simulink model "roll_control"  (R2020b)
settings: Solver=VariableStepAuto  StartTime=0.0  StopTime=3.45  FixedStep=0.001  RelTol=1e-5  AbsTol=1e-6
PostLoadFcn:
  | path = fileparts(which(bdroot))
  | cd(path)
  | masscgI = xlsread('mass,cg,I','mass,cg,I');
  | ThrustTable = xlsread('F15_Thrust','Sheet1');
  | u = xlsread('../../scp_new_problem/src/u.csv','u');
InitFcn:
  | HeightAboveSeaLevel = 5.4419142084;
  | 
  | GustStart = 1;
  | GustLength = [120, 130, 80];
  | GuestAmplitude = [ 2.5, -2.5,  1];
  | 
  | ShearSpeed = 4;
  | ShearDirection = 75;
  | 
  | Croll = 0.001 * (rand - 0.5);
  | Cyaw = 0.05 * (rand - 0.5);
  | Cside = 0.001 * (rand - 0.5);
  | 
  | GustStart = 2 * rand;
  | GustLength = [100 + 50 * (rand - 0.5), 100 + 50 * (rand - 0.5), 100 + 50 * (rand - 0.5)];
  | GuestAmplitude = [ 5 * (rand - 0.5), 5 * (rand - 0.5),  5 * (rand - 0.5)];
  | 
  | ShearSpeed = 5 * rand;
  | ShearDirection = 360 * rand;
  | 
  | HeightAboveSeaLevel = rand * 1000;
values from neighbouring files (symbols this model uses):
  cg = temp(4)    [NonlinearStateEstimationForActuatorDelay.m]
  D = zeros(size(B))    [RocketOutputFunction.m]    (also in StateSpaceController.m; TimeDelayCompensationElevator.m = [0; 0])
  F = eye(6)    [MEKFAttitudeOnly.m]
  I = reshape(x(1:9), [3 3])    [AdaptiveLQR.m]    (also in MEKF.m = diag([0.08 0.08 0.002]); MEKFAttitudeOnly.m = diag([0.08 0.08 0.002]); MEKF_old.m = diag([0.08 0.08 0.002]); NonlinearStateEstimationForActuatorDelay.m = diag([Ixx, Ixx, Izz]))
  K = 1.1    [DATCOMvsOR.m]    (also in Forces_and_Moments_Calculator.m; MEKF.m = (P * H.') / (H * P * H.' + V); MEKFAttitudeOnly.m = P2 * H' * inv(S); MEKF_old.m = (P * H.') / (H * P * H.' + V))
  mass = 1.0565    [ImpactVelocityNotParallelMatlab.m]    (also in NonlinearStateEstimationForActuatorDelay.m = temp(1); OneDLanding.m; RunImpactVelocityParforCompiled.m; StateSpaceController.m = 1.0616753546)
  q = x(13:16)    [AdaptiveLQR.m]    (also in MEKF.m = nominal_state(4:7); MEKFAttitudeOnly.m = [1 0 0 0]; MEKF_old.m = nominal_state(4:7); NonlinearStateEstimationForActuatorDelay.m = x(4:7))
  r = [0; 0; -(rocket_length - Average_cg)]    [StateSpaceController.m]    (also in TimeDelayCompensationElevator.m = [0;0]; Tracker.m)
  s = linspace(0, 100, nums)    [ImpactVelocityFunction.m]    (also in ImpactVelocityNotParallelMatlab.m = 1:5:500; ParallelImpactVelocity.m = .1:.01:500; ParralelRun.m = linspace(5,7, nums); RunImpactVelocityParforCompiled.m = 1:0.1:500)
  whentoignite = [s(row); v(col)]    [SecondPartLandingAlgorithm.m]
undefined symbols (not defined in the file or in its folder): Angle, Axis, deg, e0_0, e1_0, e2_0, e3_0, Earth, Kri, Light, magnitude, MIL, rad, WGS84
libraries: aerolibutil x7, vrlib x6, shared6dof x6, aerolibconvert2 x5, simulink x4, sharedtransform x4, aerolibwind2 x3, pid_lib x3, robotcorelib x2, sharedutil x2, aerolibasang x2, aerolibatmos2 x1
(part 2 of 3)

== system roll_control/Subsystem/Acceleration Calculator/Aero Forces and Moments ==
  Mach : Inport
  Local Airspeed (m/s) : Inport  Port=2
  AoA (rad) : Inport  Port=3
  Density : Inport  Port=4
  Temperature : Inport  Port=5
  Dynamic Pressure : Inport  Port=6
  Center of Mass X : Inport  Port=7
  Angular velocity (rad/s) : Inport  Port=8
  Axial Drag Calculator : Subsystem
  CN and Cm calculator : Subsystem
  Coefficients to Force : Subsystem
  Coefficients to Moment : Subsystem
  Constants : Subsystem
  Croll : Constant  Value=Croll
  Cside : Constant  Value=Cside
  Cyaw : Constant  Value=Cyaw
  Dynamic Pressure * Ref Area : Product
  Theta Rotation : Subsystem
  Aero Forces (N) : Outport  VectorParamsAs1DForOutWhenUnconnected=off
  Aero Moments (Nm) : Outport  Port=2  VectorParamsAs1DForOutWhenUnconnected=off
  wires:
  AoA (rad)/1 -> Axial Drag Calculator/2(AoA (rad)), CN and Cm calculator/3(AoA (rads))
  Temperature/1 -> Axial Drag Calculator/4(Temperature)
  Coefficients to Force/1(Force (N)) -> Aero Forces (N)/1
  Mach/1 -> Axial Drag Calculator/1(Mach), CN and Cm calculator/1(Mach)
  CN and Cm calculator/1(CN) -> Coefficients to Force/3(CN)
  Angular velocity (rad/s)/1 -> CN and Cm calculator/5(Angular Velocity (rad/s))
  Center of Mass X/1 -> CN and Cm calculator/4(Center of Mass X)
  Axial Drag Calculator/1(Caxial) -> Coefficients to Force/1(Caxial)
  Dynamic Pressure/1 -> Dynamic Pressure * Ref Area/1
  Local Airspeed (m/s)/1 -> Axial Drag Calculator/13(Airspeed), CN and Cm calculator/2(Airspeed (m/s)), Theta Rotation/1(Local Airspeed (m/s))
  Cside/1 -> Coefficients to Force/2(Cside)
  Coefficients to Moment/1(Moments (Nm)) -> Aero Moments (Nm)/1
  CN and Cm calculator/2(Cm) -> Coefficients to Moment/4(Cpitch)
  Theta Rotation/1(Theta Rotation Matrix) -> Coefficients to Moment/2(Theta Rotation Matrix), Coefficients to Force/4(Theta Rotation), CN and Cm calculator/6(Theta Rotation Matrix)
  Dynamic Pressure * Ref Area/1 -> Coefficients to Force/5(z), Coefficients to Moment/1(z)
  Constants/1(Reference diameter (m)) -> CN and Cm calculator/7(Reference Diameter (m)), Coefficients to Moment/5(Reference Diameter (m))
  Constants/3(Reference area (m^2)) -> Dynamic Pressure * Ref Area/2, CN and Cm calculator/8(Reference Area (m^2)), Axial Drag Calculator/9(Reference Area (m^2))
  Constants/4(Nose Cone Length (m)) -> Axial Drag Calculator/10(Nose Cone Length (m)), CN and Cm calculator/9(Nose Cone Length (m))
  Constants/5(Body Tube Length (m)) -> Axial Drag Calculator/5(Body Tube Length (m)), CN and Cm calculator/10(Body Tube Length (m))
  Constants/8(Nose Cone Planform Area (m^2)) -> CN and Cm calculator/11(Nose Cone Planform Area (m^2))
  Constants/9(Body Tube Planform Area (m^2)) -> CN and Cm calculator/12(Body Tube Planform Area (m^2))
  Constants/12(Body Tube CP (m)) -> CN and Cm calculator/13(Body Tube CP)
  Constants/13(Nose Cone CP (m)) -> CN and Cm calculator/14(Nose Cone CP)
  Constants/14(Pitch Center X (m)) -> CN and Cm calculator/15(Pitch Center X)
  Constants/7(Body Tube Wet Area (m^2)) -> Axial Drag Calculator/6(Body Tube Wet Area (m^2))
  Constants/6("Nose Cone Wet Area (m^2) ") -> Axial Drag Calculator/7(Nose Cone Wet Area (m^2))
  Constants/2(Reference radius (m)) -> Axial Drag Calculator/8(Reference Radius (m))
  Constants/10(Surface Roughness (m)) -> Axial Drag Calculator/11(Surface Roughness)
  Constants/11(sin(phi)) -> Axial Drag Calculator/12(sinphi)
  Density/1 -> Axial Drag Calculator/3(Density)
  Cyaw/1 -> Coefficients to Moment/3(Cyaw)
  Croll/1 -> Coefficients to Moment/6(Croll)

== system roll_control/Subsystem/Acceleration Calculator/Check if Height is 0 ==
  Force : Inport
  Moments : Inport  Port=2
  Xe (m) : Inport  Port=3
  0,3 : Constant  Value=[0;0;0]
  1 : Constant  Value=[0 0]
  2 : Constant  Value=0
  Height : Selector  InputPortWidth=3  IndexOptions=Index vector (dialog)  Indices=3  OutputSizes=1
  If on ground : Switch  Criteria=u2 > Threshold
  If on ground and force is not up : Switch  Criteria=u2 > Threshold
  Mux : Mux  Inputs=2
  Selector : Selector  InputPortWidth=3  IndexOptions=Index vector (dialog)  Indices=3  OutputSizes=1
  mul3 : Switch  Criteria=u2 ~= 0  Threshold=deg2rad(17)
  Force (N) : Outport  VectorParamsAs1DForOutWhenUnconnected=off
  Moments (Nm) : Outport  Port=2  VectorParamsAs1DForOutWhenUnconnected=off
  wires:
  Moments/1 -> mul3/1
  Force/1 -> If on ground/1, Selector/1
  Xe (m)/1 -> Height/1
  0,3/1 -> mul3/3
  Height/1 -> If on ground/2, mul3/2
  2/1 -> If on ground and force is not up/3
  Selector/1 -> If on ground and force is not up/1, If on ground and force is not up/2
  1/1 -> Mux/1
  Mux/1 -> If on ground/3
  If on ground and force is not up/1 -> Mux/2
  If on ground/1 -> Force (N)/1
  mul3/1 -> Moments (Nm)/1

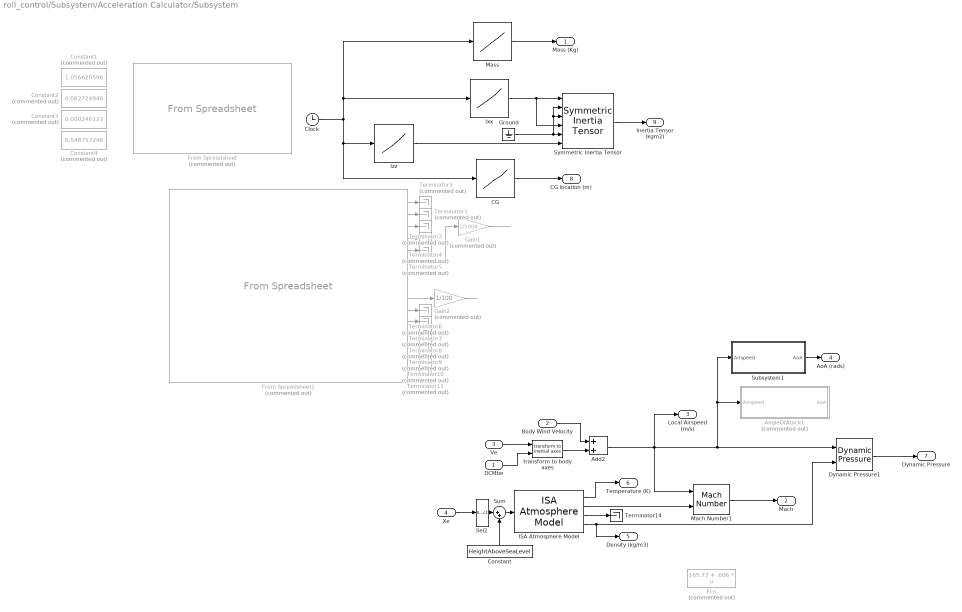
== system roll_control/Subsystem/Acceleration Calculator/Subsystem ==
  DCMbe : Inport
  Body Wind Velocity : Inport  Port=2
  Ve : Inport  Port=3
  Xe : Inport  Port=4
  Add2 : Sum
  AngleOfAtack1 : MATLAB Function  Commented=on  TreatAsAtomicUnit=on
  CG : Lookup_n-D  NumberOfTableDimensions=1  BreakpointsForDimension1=masscgI(:,1)  BreakpointsForDimension1FirstPoint=0  BreakpointsForDimension1Spacing=1.5e-5  Table=masscgI(:,5)  ExtrapMethod=Clip  InternalRulePriority=Speed  RndMeth=Simplest  InputSameDT=on
  Clock : Clock
  Constant : Constant  Value=HeightAboveSeaLevel
  Constant1 : Constant  Commented=on  Value=1.056620596
  Constant2 : Constant  Commented=on  Value=0.082724946
  Constant3 : Constant  Commented=on  Value=0.000246123
  Constant4 : Constant  Commented=on  Value=0.548757246
  Dynamic Pressure1 : aerolibasang/Dynamic Pressure
  Fcn : Fcn  Commented=on  Expr=165.77 + .606 * u
  From Spreadsheet : FromSpreadsheet  Commented=on  FileName=mass,cg,I.xlsx  SheetName=mass,cg,I  Range=A1:E4395  ExtrapolationBeforeFirstDataPoint=Hold first value  InterpolationWithinTimeRange=Zero order hold  ExtrapolationAfterLastDataPoint=Hold last value
  From Spreadsheet1 : FromSpreadsheet  Commented=on  FileName=cg mass MOI.xlsx  SheetName=cg mass MOI  Range=A1:E4395  ExtrapolationBeforeFirstDataPoint=Hold first value  ExtrapolationAfterLastDataPoint=Hold last value
  Gain1 : Gain  Commented=on  Gain=1/1000
  Gain2 : Gain  Commented=on  Gain=1/100
  Ground : Ground
  ISA Atmosphere Model : aerolibatmos2/ISA Atmosphere Model  custom=on  g=9.80665  gamma=1.4  R=287.0531  L=0.0065  h_trop=11000  h_strat=20000  rho0=1.225  P0=101325  T0=288.15  h0=0
  Ixx : Lookup_n-D  NumberOfTableDimensions=1  BreakpointsForDimension1=masscgI(:,1)  BreakpointsForDimension1FirstPoint=0  BreakpointsForDimension1Spacing=1.5e-5  Table=masscgI(:,3)  ExtrapMethod=Clip  InternalRulePriority=Speed  RndMeth=Simplest  InputSameDT=on
  Izz : Lookup_n-D  NumberOfTableDimensions=1  BreakpointsForDimension1=masscgI(:,1)  BreakpointsForDimension1FirstPoint=0  BreakpointsForDimension1Spacing=1.5e-5  Table=masscgI(:,4)  ExtrapMethod=Clip  InternalRulePriority=Speed  RndMeth=Simplest  InputSameDT=on
  Mach Number1 : aerolibasang/Mach Number
      settings: SourceProductBaseCode=AE
  Mass : Lookup_n-D  NumberOfTableDimensions=1  BreakpointsForDimension1=masscgI(:,1)  BreakpointsForDimension1FirstPoint=0  BreakpointsForDimension1Spacing=1.5e-5  Table=masscgI(:,2)  ExtrapMethod=Clip  InternalRulePriority=Speed  RndMeth=Simplest  InputSameDT=on
  Sel2 : Selector  InputPortWidth=3  IndexOptions=Index vector (dialog)  Indices=3  OutputSizes=1
  Subsystem1 : Subsystem
  Sum : Sum  Inputs=|++
  Symmetric Inertia Tensor : aerolibbdyn/Symmetric Inertia Tensor
      settings: SourceProductBaseCode=AE
  Terminator{1..11} (11 alike) : Terminator  Commented=on
  Terminator14 : Terminator
  "transform to body axes " : shared6dof/6DOF (Euler Angles)/transform to Inertial axes   SystemSampleTime=-1  VariantActivationTime=update diagram  Latency=0  AutoFrameSizeCalculation=off
      settings: SourceProductBaseCode=AE,PW,MT,UV,VE,VP
  Mass (Kg) : Outport  VectorParamsAs1DForOutWhenUnconnected=off
  Mach : Outport  Port=2  VectorParamsAs1DForOutWhenUnconnected=off
  Local Airspeed (m/s) : Outport  Port=3  VectorParamsAs1DForOutWhenUnconnected=off
  AoA (rads) : Outport  Port=4  VectorParamsAs1DForOutWhenUnconnected=off
  Density (kg/m3) : Outport  Port=5  VectorParamsAs1DForOutWhenUnconnected=off
  Temperature (K) : Outport  Port=6  VectorParamsAs1DForOutWhenUnconnected=off
  Dynamic Pressure : Outport  Port=7  VectorParamsAs1DForOutWhenUnconnected=off
  CG location (m) : Outport  Port=8  VectorParamsAs1DForOutWhenUnconnected=off
  Inertia Tensor (kgm2) : Outport  Port=9  VectorParamsAs1DForOutWhenUnconnected=off
  wires:
  From Spreadsheet1/4 -> Terminator4/1
  ISA Atmosphere Model/4 -> Density (kg/m3)/1, Dynamic Pressure1/2
  From Spreadsheet1/5 -> Terminator5/1
  From Spreadsheet1/9 -> Gain2/1
  From Spreadsheet1/6 -> Gain1/1
  Dynamic Pressure1/1 -> Dynamic Pressure/1
  Mach Number1/1 -> Mach/1
  From Spreadsheet1/12 -> Terminator8/1
  ISA Atmosphere Model/3 -> Terminator14/1
  Gain2/1 -> ?
  From Spreadsheet1/11 -> Terminator7/1
  Xe/1 -> Sel2/1
  From Spreadsheet1/3 -> Terminator2/1
  From Spreadsheet1/14 -> Terminator10/1
  From Spreadsheet1/2 -> Terminator1/1
  From Spreadsheet1/1 -> Terminator3/1
  From Spreadsheet1/13 -> Terminator9/1
  From Spreadsheet1/15 -> Terminator11/1
  Gain1/1 -> ?
  Ground/1 -> Symmetric Inertia Tensor/2, Symmetric Inertia Tensor/3, Symmetric Inertia Tensor/5
  Symmetric Inertia Tensor/1 -> Inertia Tensor (kgm2)/1
  From Spreadsheet1/10 -> Terminator6/1
  Sel2/1 -> Sum/1
  Ve/1 -> "transform to body axes "/1
  DCMbe/1 -> "transform to body axes "/2
  Add2/1 -> Local Airspeed (m/s)/1, Subsystem1/1(Airspeed), AngleOfAtack1/1(Airspeed), Dynamic Pressure1/1, Mach Number1/1
  Subsystem1/1(AoA) -> AoA (rads)/1
  "transform to body axes "/1 -> Add2/2
  Clock/1 -> Izz/1, CG/1, Ixx/1, Mass/1
  Body Wind Velocity/1 -> Add2/1
  ISA Atmosphere Model/1 -> Temperature (K)/1
  ISA Atmosphere Model/2 -> Mach Number1/2
  Mass/1 -> Mass (Kg)/1
  Ixx/1 -> Symmetric Inertia Tensor/4, Symmetric Inertia Tensor/1
  Izz/1 -> Symmetric Inertia Tensor/6
  CG/1 -> CG location (m)/1
  Sum/1 -> ISA Atmosphere Model/1
  Constant/1 -> Sum/2

== system roll_control/Subsystem/Subsystem1/Subsystem ==
  p q r : Inport
  Constant9 : Constant  Commented=on  Value=[0.99^.5 0.1 0 0]
  Initial Euler Angles : Constant  Value=[0 0 0]
  Quaternion Normalize : sharedutil/Quaternion Normalize  aMode=aMode
      settings: SourceProductBaseCode=AE,PW,MT,UV,VE,VP
  Quaternions to Direction Cosine Matrix : sharedtransform/Quaternions to  Direction Cosine Matrix  aMode=aMode
      settings: SourceProductBaseCode=AE,PW,MT,UV,VE,VP
  Quaternions to Rotation Angles : sharedtransform/Quaternions to Rotation Angles  rotationOrder=ZYX  aMode=aMode
      settings: SourceProductBaseCode=AE,PW,MT,UV,VE,VP
  Rotation Angles to Quaternions : sharedtransform/Rotation Angles to Quaternions  rotationOrder=ZYX  aMode=aMode
      settings: SourceProductBaseCode=AE,PW,MT,UV,VE,VP
  Selector : Selector  IndexMode=Zero-based  InputPortWidth=3  IndexOptions=Index vector (dialog)  Indices=[ 2 1 0]  OutputSizes=1
  Selector1 : Selector  IndexMode=Zero-based  InputPortWidth=3  IndexOptions=Index vector (dialog)  Indices=[2 1 0]  OutputSizes=1
  Subsystem : Subsystem
  q0 q1 q2 q3 : Integrator  InitialConditionSource=external  InitialCondition=[e0_0 e1_0 e2_0 e3_0]
  DCM : Outport  VectorParamsAs1DForOutWhenUnconnected=off
  Euler : Outport  Port=2  VectorParamsAs1DForOutWhenUnconnected=off
  Quaternion : Outport  Port=3  VectorParamsAs1DForOutWhenUnconnected=off
  wires:
  Selector/1 -> Euler/1
  Initial Euler Angles/1 -> Selector1/1
  Selector1/1 -> Rotation Angles to Quaternions/1
  q0 q1 q2 q3/1 -> Quaternion Normalize/1
  Quaternions to Direction Cosine Matrix/1 -> DCM/1
  Subsystem/1(qdot1) -> q0 q1 q2 q3/1
  p q r/1 -> Subsystem/1(p q r1)
  Quaternions to Rotation Angles/1 -> Selector/1
  Quaternion Normalize/1 -> Quaternion/1, Subsystem/2(q0 q1 q2 q1), Quaternions to Rotation Angles/1, Quaternions to Direction Cosine Matrix/1
  Rotation Angles to Quaternions/1 -> q0 q1 q2 q3/2
  Constant9/1 -> ?

== system roll_control/Subsystem/Wind/Subsystem3 ==
  Rocket velocity (m/s) Ve : Inport
  height (m) : Inport  Port=2
  DCMbe : Inport  Port=3
  Discrete Wind Gust Model : aerolibwind2/Discrete Wind Gust Model  units=Metric (MKS)  Gx=on  Gy=on  Gz=on  t_0=GustStart  d_m=GustLength  v_m=GuestAmplitude
  Dot Product : DotProduct  SaturateOnIntegerOverflow=on  OutDataTypeStr=Inherit: Inherit via internal rule
  Sum : Sum  Inputs=3
  V : Math  Operator=sqrt  SignedPower=on  SaturateOnIntegerOverflow=on
  Von Karman Wind Turbulence Model (Continuous (+q +r)) : aerolibwind2/Dryden Wind Turbulence Model  (Continuous (+q -r))  units=Metric (MKS)  spec=MIL-F-8785C  model=Discrete Dryden (+q -r)  W20=ShearSpeed  Wdeg=ShearDirection  TurbProb=10^-2 - Light  L_high=762  Wingspan=1  ts=0.1  Seed=[23341 23342 23343 23344]  T_on=on
  Wind Shear Model : aerolibwind2/Wind Shear Model  units=Metric (MKS)  phase=Category C - Terminal Flight Phase  W_20=ShearSpeed  Wdeg=ShearDirection
  wind angular velocity (rad/s) : Outport  VectorParamsAs1DForOutWhenUnconnected=off
  body axis wind velocity (m/s) : Outport  Port=2  VectorParamsAs1DForOutWhenUnconnected=off
  wires:
  height (m)/1 -> Wind Shear Model/1, Von Karman Wind Turbulence Model (Continuous (+q +r))/1
  Discrete Wind Gust Model/1 -> Sum/1
  DCMbe/1 -> Wind Shear Model/2, Von Karman Wind Turbulence Model (Continuous (+q +r))/3
  V/1 -> Von Karman Wind Turbulence Model (Continuous (+q +r))/2, Discrete Wind Gust Model/1
  Sum/1 -> body axis wind velocity (m/s)/1
  Wind Shear Model/1 -> Sum/3
  Von Karman Wind Turbulence Model (Continuous (+q +r))/1 -> Sum/2
  Von Karman Wind Turbulence Model (Continuous (+q +r))/2 -> wind angular velocity (rad/s)/1
  Dot Product/1 -> V/1
  Rocket velocity (m/s) Ve/1 -> Dot Product/1, Dot Product/2

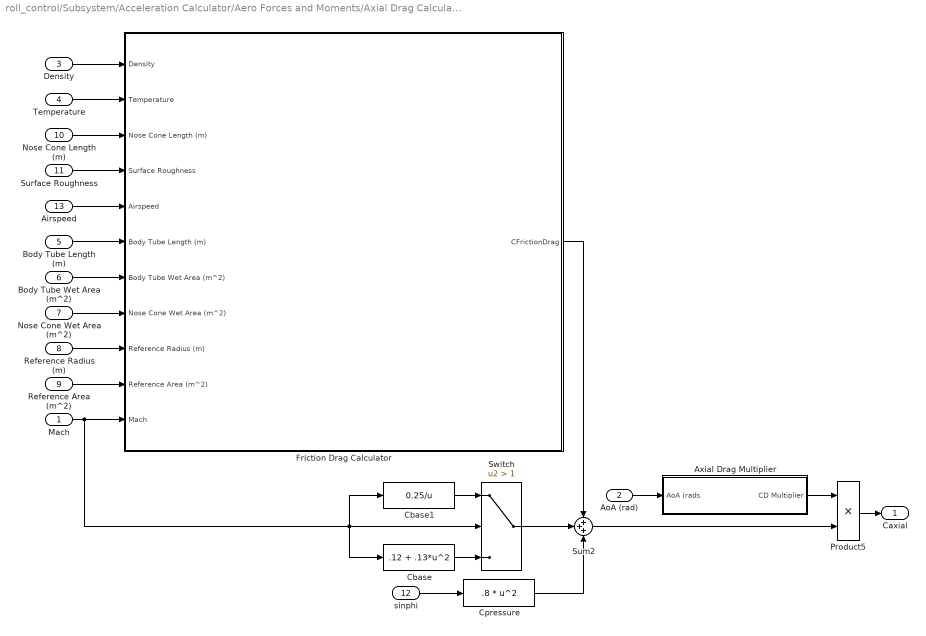
== system roll_control/Subsystem/Acceleration Calculator/Aero Forces and Moments/Axial Drag Calculator ==
  Mach : Inport
  AoA (rad) : Inport  Port=2
  Density : Inport  Port=3
  Temperature : Inport  Port=4
  Body Tube Length (m) : Inport  Port=5
  Body Tube Wet Area (m^2) : Inport  Port=6
  Nose Cone Wet Area (m^2) : Inport  Port=7
  Reference Radius (m) : Inport  Port=8
  Reference Area (m^2) : Inport  Port=9
  Nose Cone Length (m) : Inport  Port=10
  Surface Roughness : Inport  Port=11
  sinphi : Inport  Port=12
  Airspeed : Inport  Port=13
  Axial Drag Multiplier : Subsystem
  Cbase : Fcn  Expr=.12 + .13*u^2
  Cbase1 : Fcn  Expr=0.25/u
  Cpressure : Fcn  Expr=.8 * u^2
  Friction Drag Calculator : Subsystem
  Product5 : Product
  Sum2 : Sum  Inputs=+++
  Switch : Switch  Criteria=u2 > Threshold  Threshold=1
  Caxial : Outport  VectorParamsAs1DForOutWhenUnconnected=off
  wires:
  Nose Cone Wet Area (m^2)/1 -> Friction Drag Calculator/8(Nose Cone Wet Area (m^2))
  Reference Area (m^2)/1 -> Friction Drag Calculator/10(Reference Area (m^2))
  Reference Radius (m)/1 -> Friction Drag Calculator/9(Reference Radius (m))
  Body Tube Wet Area (m^2)/1 -> Friction Drag Calculator/7(Body Tube Wet Area (m^2))
  sinphi/1 -> Cpressure/1
  Airspeed/1 -> Friction Drag Calculator/5(Airspeed)
  Surface Roughness/1 -> Friction Drag Calculator/4(Surface Roughness)
  Temperature/1 -> Friction Drag Calculator/2(Temperature)
  Mach/1 -> Cbase/1, Cbase1/1, Switch/2, Friction Drag Calculator/11(Mach)
  Density/1 -> Friction Drag Calculator/1(Density)
  Nose Cone Length (m)/1 -> Friction Drag Calculator/3(Nose Cone Length (m))
  Body Tube Length (m)/1 -> Friction Drag Calculator/6(Body Tube Length (m))
  Product5/1 -> Caxial/1
  Friction Drag Calculator/1(CFrictionDrag) -> Sum2/1
  Cbase/1 -> Switch/3
  Cpressure/1 -> Sum2/3
  AoA (rad)/1 -> Axial Drag Multiplier/1(AoA (rads)
  Sum2/1 -> Product5/2
  Axial Drag Multiplier/1(CD Multiplier) -> Product5/1
  Cbase1/1 -> Switch/1
  Switch/1 -> Sum2/2

== system roll_control/Subsystem/Acceleration Calculator/Aero Forces and Moments/CN and Cm calculator ==
  Mach : Inport
  Airspeed (m/s) : Inport  Port=2
  AoA (rads) : Inport  Port=3
  Center of Mass X : Inport  Port=4
  Angular Velocity (rad/s) : Inport  Port=5
  Theta Rotation Matrix : Inport  Port=6
  Reference Diameter (m) : Inport  Port=7
  Reference Area (m^2) : Inport  Port=8
  Nose Cone Length (m) : Inport  Port=9
  Body Tube Length (m) : Inport  Port=10
  Nose Cone Planform Area (m^2) : Inport  Port=11
  Body Tube Planform Area (m^2) : Inport  Port=12
  Body Tube CP : Inport  Port=13
  Nose Cone CP : Inport  Port=14
  Pitch Center X : Inport  Port=15
  CM calculator : Subsystem
  CN calculator : Subsystem
  CN : Outport  VectorParamsAs1DForOutWhenUnconnected=off
  Cm : Outport  Port=2  VectorParamsAs1DForOutWhenUnconnected=off
  wires:
  Body Tube Planform Area (m^2)/1 -> CM calculator/14(Body Tube Planform Area (m^2)), CN calculator/5(Body Tube Planform Area (m^2))
  Pitch Center X/1 -> CM calculator/8(Pitch Center X)
  Nose Cone CP/1 -> CM calculator/5(Nose Cone CP)
  Body Tube CP/1 -> CM calculator/4(Body Tube CP)
  Nose Cone Planform Area (m^2)/1 -> CM calculator/13(Nose Cone Planform Area (m^2)), CN calculator/4(Nose Cone Planform Area (m^2))
  Angular Velocity (rad/s)/1 -> CM calculator/2(Angular Velocity (rad/s))
  Reference Area (m^2)/1 -> CN calculator/1(Reference Area (m^2)), CM calculator/6(Reference Area (m^2))
  AoA (rads)/1 -> CN calculator/2(AoA (rads))
  Mach/1 -> CN calculator/3(Mach)
  Center of Mass X/1 -> CM calculator/7(Center of Mass X)
  CN calculator/3(CN) -> CN/1, CM calculator/11(CN)
  CN calculator/2(Body Tube CN) -> CM calculator/10(Body Tube CN)
  CN calculator/1(Nose Cone CN) -> CM calculator/9(Nose Cone CN)
  Airspeed (m/s)/1 -> CM calculator/1(Airspeed (m/s))
  Theta Rotation Matrix/1 -> CM calculator/3(Theta Rotation Matrix)
  Reference Diameter (m)/1 -> CM calculator/12(Reference Diameter (m))
  Nose Cone Length (m)/1 -> CM calculator/15(Nose Cone Length (m))
  CM calculator/1(Cm) -> Cm/1
  Body Tube Length (m)/1 -> CM calculator/16(Body Tube Length (m))

== system roll_control/Subsystem/Acceleration Calculator/Aero Forces and Moments/Coefficients to Force ==
  Caxial : Inport
  Cside : Inport  Port=2
  CN : Inport  Port=3
  Theta Rotation : Inport  Port=4
  z : Inport  Port=5
  Aero Forces : Product  Inputs=**  Multiplication=Matrix(*)
  Gain5 : Gain  Gain=-1
  Multiply : Product
  Vector Concatenate3 : Concatenate  NumInputs=3
  Force (N) : Outport  VectorParamsAs1DForOutWhenUnconnected=off
  wires:
  Vector Concatenate3/1 -> Gain5/1
  Gain5/1 -> Multiply/2
  Caxial/1 -> Vector Concatenate3/3
  CN/1 -> Vector Concatenate3/1
  Multiply/1 -> Aero Forces/2
  Aero Forces/1 -> Force (N)/1
  Theta Rotation/1 -> Aero Forces/1
  Cside/1 -> Vector Concatenate3/2
  z/1 -> Multiply/1

== system roll_control/Subsystem/Acceleration Calculator/Aero Forces and Moments/Coefficients to Moment ==
  z : Inport
  Theta Rotation Matrix : Inport  Port=2
  Cyaw : Inport  Port=3
  Cpitch : Inport  Port=4
  Reference Diameter (m) : Inport  Port=5
  Croll : Inport  Port=6
  Aero Moments : Product  Inputs=**  Multiplication=Matrix(*)
  CNCMxL1 : Product  Inputs=***
  Gain4 : Gain  Gain=-1
  Vector Concatenate4 : Concatenate  NumInputs=3
  Moments (Nm) : Outport  VectorParamsAs1DForOutWhenUnconnected=off
  wires:
  Gain4/1 -> Vector Concatenate4/1
  Vector Concatenate4/1 -> CNCMxL1/2
  Reference Diameter (m)/1 -> CNCMxL1/3
  CNCMxL1/1 -> Aero Moments/2
  Cyaw/1 -> Gain4/1
  Croll/1 -> Vector Concatenate4/3
  z/1 -> CNCMxL1/1
  Theta Rotation Matrix/1 -> Aero Moments/1
  Cpitch/1 -> Vector Concatenate4/2
  Aero Moments/1 -> Moments (Nm)/1

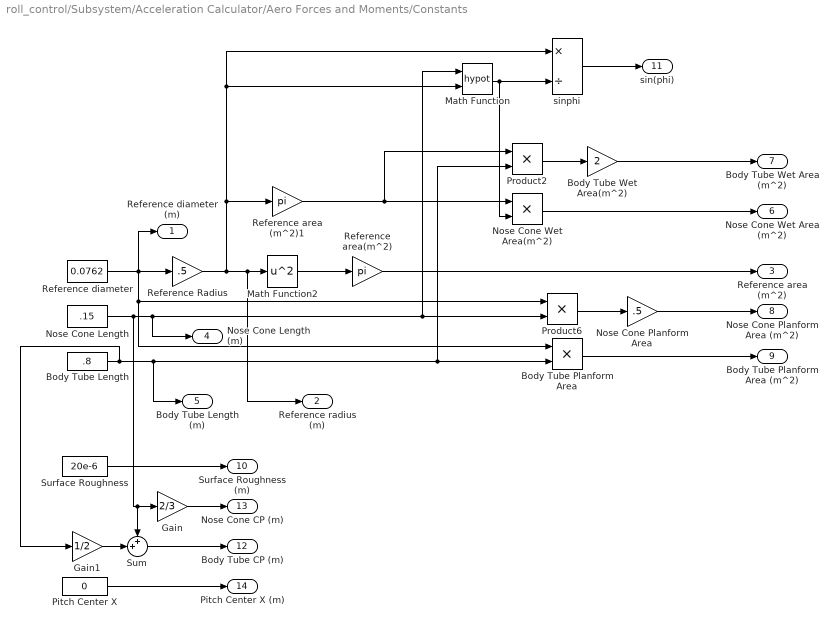
== system roll_control/Subsystem/Acceleration Calculator/Aero Forces and Moments/Constants ==
  Body Tube Length : Constant  Value=.8
  Body Tube Planform Area : Product
  Body Tube Wet Area(m^2) : Gain  Gain=2
  Gain : Gain  Gain=2/3
  Gain1 : Gain  Gain=1/2
  Math Function : Math  Operator=hypot  SignedPower=on  SaturateOnIntegerOverflow=on
  Math Function2 : Math  Operator=square  SignedPower=on  SaturateOnIntegerOverflow=on
  Nose Cone Length : Constant  Value=.15
  Nose Cone Planform Area : Gain  Gain=.5
  Nose Cone Wet Area(m^2) : Product
  Pitch Center X : Constant  Value=0
  Product2 : Product
  Product6 : Product
  Reference Radius : Gain  Gain=.5
  Reference area (m^2)1 : Gain  Gain=pi
  Reference area(m^2) : Gain  Gain=pi
  Reference diameter : Constant  Value=0.0762
  Sum : Sum  Inputs=++|
  Surface Roughness : Constant  Value=20e-6
  sinphi : Product  Inputs=*/
  Reference diameter (m) : Outport  VectorParamsAs1DForOutWhenUnconnected=off
  Reference radius (m) : Outport  Port=2  VectorParamsAs1DForOutWhenUnconnected=off
  Reference area (m^2) : Outport  Port=3  VectorParamsAs1DForOutWhenUnconnected=off
  Nose Cone Length (m) : Outport  Port=4  VectorParamsAs1DForOutWhenUnconnected=off
  Body Tube Length (m) : Outport  Port=5  VectorParamsAs1DForOutWhenUnconnected=off
  "Nose Cone Wet Area (m^2) " : Outport  Port=6  VectorParamsAs1DForOutWhenUnconnected=off
  Body Tube Wet Area (m^2) : Outport  Port=7  VectorParamsAs1DForOutWhenUnconnected=off
  Nose Cone Planform Area (m^2) : Outport  Port=8  VectorParamsAs1DForOutWhenUnconnected=off
  Body Tube Planform Area (m^2) : Outport  Port=9  VectorParamsAs1DForOutWhenUnconnected=off
  Surface Roughness (m) : Outport  Port=10  VectorParamsAs1DForOutWhenUnconnected=off
  sin(phi) : Outport  Port=11  VectorParamsAs1DForOutWhenUnconnected=off
  Body Tube CP (m) : Outport  Port=12  VectorParamsAs1DForOutWhenUnconnected=off
  Nose Cone CP (m) : Outport  Port=13  VectorParamsAs1DForOutWhenUnconnected=off
  Pitch Center X (m) : Outport  Port=14  VectorParamsAs1DForOutWhenUnconnected=off
  wires:
  Reference diameter/1 -> Reference diameter (m)/1, Body Tube Planform Area/1, Product6/1, Reference Radius/1
  Math Function2/1 -> Reference area(m^2)/1
  Nose Cone Length/1 -> Product6/2, Math Function/1, Nose Cone Length (m)/1, Sum/1, Gain/1
  Product6/1 -> Nose Cone Planform Area/1
  Reference Radius/1 -> Math Function2/1, Reference radius (m)/1, Math Function/2, sinphi/1, Reference area (m^2)1/1
  Reference area (m^2)1/1 -> Product2/1, Nose Cone Wet Area(m^2)/1
  Product2/1 -> Body Tube Wet Area(m^2)/1
  Math Function/1 -> Nose Cone Wet Area(m^2)/2, sinphi/2
  Reference area(m^2)/1 -> Reference area (m^2)/1
  Nose Cone Wet Area(m^2)/1 -> "Nose Cone Wet Area (m^2) "/1
  Body Tube Wet Area(m^2)/1 -> Body Tube Wet Area (m^2)/1
  Body Tube Planform Area/1 -> Body Tube Planform Area (m^2)/1
  Nose Cone Planform Area/1 -> Nose Cone Planform Area (m^2)/1
  Surface Roughness/1 -> Surface Roughness (m)/1
  sinphi/1 -> sin(phi)/1
  Sum/1 -> Body Tube CP (m)/1
  Gain/1 -> Nose Cone CP (m)/1
  Pitch Center X/1 -> Pitch Center X (m)/1
  Gain1/1 -> Sum/2
  Body Tube Length/1 -> Gain1/1, Body Tube Length (m)/1, Body Tube Planform Area/2, Product2/2

== system roll_control/Subsystem/Acceleration Calculator/Aero Forces and Moments/Theta Rotation ==
  Local Airspeed (m/s) : Inport
  1 : Constant
  Demux : Demux  Outputs=2
  Dot Product : DotProduct  SaturateOnIntegerOverflow=on  OutDataTypeStr=Inherit: Inherit via internal rule
  Gain3 : Gain  Gain=-1
  Ground : Ground
  Theta Rotation : sharedutil/Create 3x3 Matrix  aMode=aMode
      settings: SourceProductBaseCode=AE,PW,MT,UV,VE,VP
  V : Math  Operator=sqrt  SignedPower=on  SaturateOnIntegerOverflow=on
  "cosa, sina" : Product  Inputs=*/
  xy Airspeed : Selector  InputPortWidth=3  IndexOptions=Index vector (dialog)  Indices=[1 2]  OutputSizes=1
  Theta Rotation Matrix : Outport  VectorParamsAs1DForOutWhenUnconnected=off
  wires:
  "cosa, sina"/1 -> Demux/1
  xy Airspeed/1 -> Dot Product/2, Dot Product/1, "cosa, sina"/1
  V/1 -> "cosa, sina"/2
  Demux/1 -> Theta Rotation/5, Theta Rotation/1
  1/1 -> Theta Rotation/9
  Ground/1 -> Theta Rotation/3, Theta Rotation/6, Theta Rotation/7, Theta Rotation/8
  Demux/2 -> Gain3/1, Theta Rotation/4
  Local Airspeed (m/s)/1 -> xy Airspeed/1
  Dot Product/1 -> V/1
  Gain3/1 -> Theta Rotation/2
  Theta Rotation/1 -> Theta Rotation Matrix/1

== system roll_control/Subsystem/Acceleration Calculator/Subsystem/Subsystem1 ==
  Airspeed : Inport
  Divide : Product  Inputs=*/
  Dot Product : DotProduct  SaturateOnIntegerOverflow=on  OutDataTypeStr=Inherit: Inherit via internal rule
  Sel1 : Selector  IndexMode=Zero-based  InputPortWidth=3  IndexOptions=Index vector (dialog)  Indices=2  OutputSizes=1
  Trigonometric Function : Trigonometry  Operator=acos
  V : Math  Operator=sqrt  SignedPower=on  SaturateOnIntegerOverflow=on
  AoA : Outport  VectorParamsAs1DForOutWhenUnconnected=off
  wires:
  Trigonometric Function/1 -> AoA/1
  Airspeed/1 -> Sel1/1, Dot Product/1, Dot Product/2
  Divide/1 -> Trigonometric Function/1
  Sel1/1 -> Divide/1
  Dot Product/1 -> V/1
  V/1 -> Divide/2

== system roll_control/Subsystem/Subsystem1/Subsystem/Subsystem ==
  p q r1 : Inport
  q0 q1 q2 q1 : Inport  Port=2
  Constant : Constant
  Dot Product : DotProduct  OutDataTypeStr=Inherit: Inherit via internal rule
  High Gain Quaternion Normalization : Gain  SaturateOnIntegerOverflow=on  OutDataTypeStr=Inherit: Same as input  ParamDataTypeStr=Inherit: Same as input
  Mux1 : Mux  Inputs=[3 4 1]
  Mux2 : Mux
  Sum : Sum  Inputs=|+-  InputSameDT=on  SaturateOnIntegerOverflow=on  OutDataTypeStr=Inherit: Same as first input
  q0dot : Fcn  Expr=-0.5 * ( u[5]*u[1]+u[6]*u[2]+u[7]*u[3] ) + u[8]*u[4]
  q1dot : Fcn  Expr=0.5 * ( u[4]*u[1]+u[6]*u[3]-u[7]*u[2] ) + u[8]*u[5]
  q2dot : Fcn  Expr=0.5 * ( u[4]*u[2]+u[7]*u[1]-u[5]*u[3] ) + u[8]*u[6]
  q3dot : Fcn  Expr=0.5 * ( u[4]*u[3]+u[5]*u[2]-u[6]*u[1] ) + u[8]*u[7]
  qdot1 : Outport  InitialOutput=0  VectorParamsAs1DForOutWhenUnconnected=off
  wires:
  Constant/1 -> Sum/1
  Dot Product/1 -> Sum/2
  Mux1/1 -> q2dot/1, q3dot/1, q0dot/1, q1dot/1
  q0 q1 q2 q1/1 -> Dot Product/1, Dot Product/2, Mux1/2
  Sum/1 -> High Gain Quaternion Normalization/1
  Mux2/1 -> qdot1/1
  q0dot/1 -> Mux2/1
  q3dot/1 -> Mux2/4
  q1dot/1 -> Mux2/2
  q2dot/1 -> Mux2/3
  High Gain Quaternion Normalization/1 -> Mux1/3
  p q r1/1 -> Mux1/1

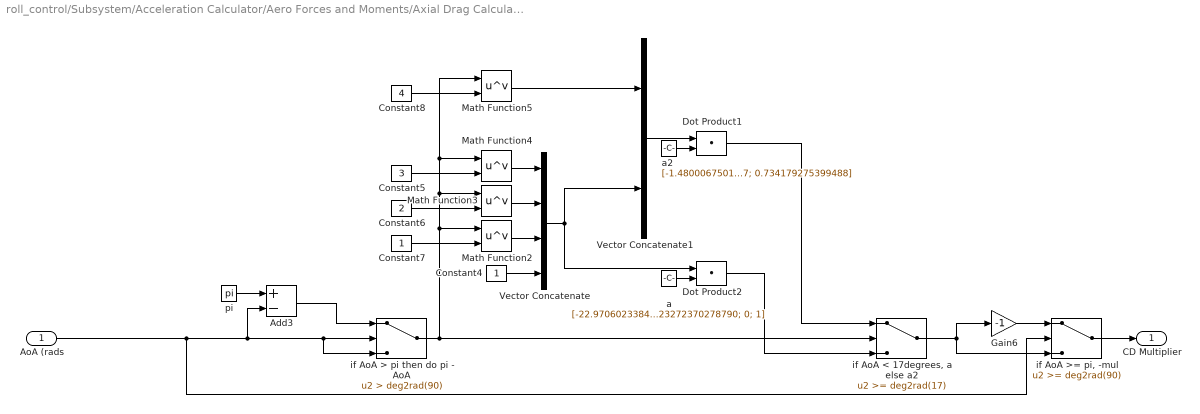
== system roll_control/Subsystem/Acceleration Calculator/Aero Forces and Moments/Axial Drag Calculator/Axial Drag Multiplier ==
  AoA (rads : Inport
  Add3 : Sum  Inputs=+-
  Constant4 : Constant
  Constant5 : Constant  Value=3
  Constant6 : Constant  Value=2
  Constant7 : Constant
  Constant8 : Constant  Value=4
  Dot Product1 : DotProduct  SaturateOnIntegerOverflow=on  OutDataTypeStr=Inherit: Inherit via internal rule
  Dot Product2 : DotProduct  SaturateOnIntegerOverflow=on  OutDataTypeStr=Inherit: Inherit via internal rule
  Gain6 : Gain  Gain=-1
  Math Function{2..5} (4 alike) : Math  Operator=pow  SignedPower=on  SaturateOnIntegerOverflow=on
  Vector Concatenate : Concatenate  NumInputs=4
  Vector Concatenate1 : Concatenate
  a : Constant  Value=[-22.970602338418825; 10.223272370278790; 0; 1]
  a2 : Constant  Value=[-1.480006750190687; 6.784940235048046; -10.062655893223173; 4.334008218595027; 0.734179275399488]
  "if AoA < 17degrees, a else a2" : Switch  Threshold=deg2rad(17)
  if AoA > pi then do pi - AoA : Switch  Criteria=u2 > Threshold  Threshold=deg2rad(90)
  "if AoA >= pi, -mul" : Switch  Threshold=deg2rad(90)
  pi : Constant  Value=pi
  CD Multiplier : Outport  VectorParamsAs1DForOutWhenUnconnected=off
  wires:
  Constant4/1 -> Vector Concatenate/4
  Constant5/1 -> Math Function4/2
  if AoA > pi then do pi - AoA/1 -> Math Function5/1, Math Function4/1, Math Function3/1, Math Function2/1, "if AoA < 17degrees, a else a2"/2
  Add3/1 -> if AoA > pi then do pi - AoA/1
  Vector Concatenate1/1 -> Dot Product1/1
  AoA (rads/1 -> "if AoA >= pi, -mul"/2, Add3/2, if AoA > pi then do pi - AoA/3, if AoA > pi then do pi - AoA/2
  a/1 -> Dot Product2/2
  "if AoA >= pi, -mul"/1 -> CD Multiplier/1
  Math Function4/1 -> Vector Concatenate/1
  "if AoA < 17degrees, a else a2"/1 -> "if AoA >= pi, -mul"/3, Gain6/1
  Gain6/1 -> "if AoA >= pi, -mul"/1
  pi/1 -> Add3/1
  Constant7/1 -> Math Function2/2
  Vector Concatenate/1 -> Vector Concatenate1/2, Dot Product2/1
  Math Function2/1 -> Vector Concatenate/3
  Constant6/1 -> Math Function3/2
  Dot Product2/1 -> "if AoA < 17degrees, a else a2"/3
  Constant8/1 -> Math Function5/2
  a2/1 -> Dot Product1/2
  Math Function5/1 -> Vector Concatenate1/1
  Math Function3/1 -> Vector Concatenate/2
  Dot Product1/1 -> "if AoA < 17degrees, a else a2"/1

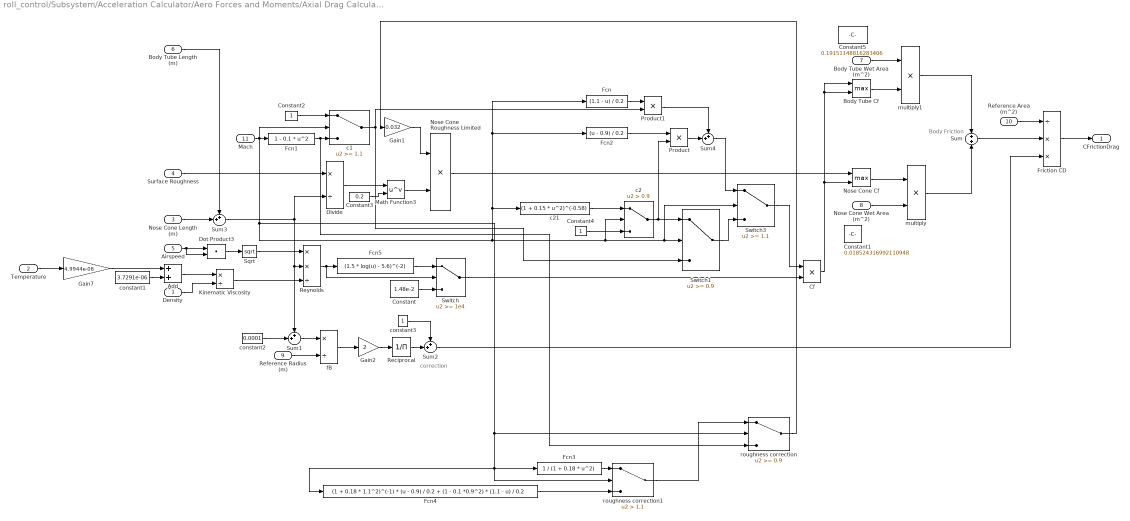
== system roll_control/Subsystem/Acceleration Calculator/Aero Forces and Moments/Axial Drag Calculator/Friction Drag Calculator ==
  note: correction
  note: Body Friction
  Density : Inport
  Temperature : Inport  Port=2
  Nose Cone Length (m) : Inport  Port=3
  Surface Roughness : Inport  Port=4
  Airspeed : Inport  Port=5
  Body Tube Length (m) : Inport  Port=6
  Body Tube Wet Area (m^2) : Inport  Port=7
  Nose Cone Wet Area (m^2) : Inport  Port=8
  Reference Radius (m) : Inport  Port=9
  Reference Area (m^2) : Inport  Port=10
  Mach : Inport  Port=11
  Add : Sum
  Body Tube Cf : MinMax  Function=max  Inputs=2
  Cf : Product  Inputs=**
  Constant : Constant  Value=1.48e-2
  Constant1 : Constant  Value=0.018524316992110948
  Constant2 : Constant
  Constant3 : Constant  Value=0.2
  Constant4 : Constant
  Constant5 : Constant  Value=0.19151148816283406
  Divide : Product  Inputs=*/
  Dot Product3 : DotProduct  SaturateOnIntegerOverflow=on  OutDataTypeStr=Inherit: Inherit via internal rule
  Fcn : Fcn  Expr=(1.1 - u) / 0.2
  Fcn1 : Fcn  Expr=1 - 0.1 * u^2
  Fcn2 : Fcn  Expr=(u - 0.9) / 0.2
  Fcn3 : Fcn  Expr=1 / (1 + 0.18 * u^2)
  Fcn4 : Fcn  Expr=(1 + 0.18 * 1.1^2)^(-1) * (u - 0.9) / 0.2 + (1 - 0.1 *0.9^2) * (1.1 - u) / 0.2
  Fcn5 : Fcn  Expr=(1.5 * log(u) - 5.6)^(-2)
  Friction CD : Product  Inputs=/**
  Gain1 : Gain  Gain=0.032
  Gain2 : Gain  Gain=2
  Gain7 : Gain  Gain=4.9944e-08
  Kinematic Viscosity : Product  Inputs=*/
  Math Function3 : Math  Operator=pow  SignedPower=on  SaturateOnIntegerOverflow=on
  Nose Cone Cf : MinMax  Function=max  Inputs=2
  Nose Cone Roughness Limited : Product  Inputs=**
  Product : Product
  Product1 : Product
  Reciprocal : Product  Inputs=/
  Reynolds : Product  Inputs=**/
  Sqrt : Sqrt  SaturateOnIntegerOverflow=on
  Sum : Sum
  Sum{1..4} (4 alike) : Sum  Inputs=++|
  Switch : Switch  Threshold=1e4
  Switch1 : Switch  Threshold=0.9
  Switch3 : Switch  Threshold=1.1
  c1 : Switch  Threshold=1.1
  c2 : Switch  Criteria=u2 > Threshold  Threshold=0.9
  c21 : Fcn  Expr=(1 + 0.15 * u^2)^(-0.58)
  constant1 : Constant  Value=3.7291e-06
  constant2 : Constant  Value=0.0001
  constant3 : Constant
  fB : Product  Inputs=*/
  multiply : Product  Inputs=**
  multiply1 : Product  Inputs=**
  roughness correction : Switch  Threshold=0.9
  roughness correction1 : Switch  Criteria=u2 > Threshold  Threshold=1.1
  CFrictionDrag : Outport  VectorParamsAs1DForOutWhenUnconnected=off
  wires:
  Sqrt/1 -> Reynolds/1
  Kinematic Viscosity/1 -> Reynolds/3
  Constant3/1 -> Math Function3/2
  constant1/1 -> Add/2
  Add/1 -> Kinematic Viscosity/1
  Gain7/1 -> Add/1
  Reynolds/1 -> Switch/2, Fcn5/1
  Gain1/1 -> Nose Cone Roughness Limited/1
  Divide/1 -> Math Function3/1
  Math Function3/1 -> Nose Cone Roughness Limited/2
  Surface Roughness/1 -> Divide/1
  Temperature/1 -> Gain7/1
  Density/1 -> Kinematic Viscosity/2
  Nose Cone Roughness Limited/1 -> Nose Cone Cf/1
  Nose Cone Length (m)/1 -> Sum3/2
  Body Tube Length (m)/1 -> Sum3/1
  Cf/1 -> Body Tube Cf/1, Body Tube Cf/2, Nose Cone Cf/2
  Nose Cone Cf/1 -> multiply/1
  Nose Cone Wet Area (m^2)/1 -> multiply/2
  Body Tube Wet Area (m^2)/1 -> multiply1/1
  Body Tube Cf/1 -> multiply1/2
  multiply/1 -> Sum/2
  multiply1/1 -> Sum/1
  constant2/1 -> Sum1/2
  Sum1/1 -> fB/1
  Reference Radius (m)/1 -> fB/2
  fB/1 -> Gain2/1
  Gain2/1 -> Reciprocal/1
  Reciprocal/1 -> Sum2/2
  constant3/1 -> Sum2/1
  Sum/1 -> Friction CD/2
  Sum2/1 -> Friction CD/3
  Reference Area (m^2)/1 -> Friction CD/1
  Friction CD/1 -> CFrictionDrag/1
  Airspeed/1 -> Dot Product3/2, Dot Product3/1
  Dot Product3/1 -> Sqrt/1
  Switch/1 -> Cf/2
  Fcn5/1 -> Switch/1
  Constant/1 -> Switch/3
  c1/1 -> Product1/2, Switch1/3
  Fcn1/1 -> roughness correction/3, c1/3
  Constant2/1 -> c1/1
  c2/1 -> Product/2, Switch1/1
  Constant4/1 -> c2/3
  c21/1 -> c2/1
  Switch3/1 -> Cf/1
  Switch1/1 -> Switch3/3
  Fcn2/1 -> Product/1
  Product/1 -> Sum4/2
  Product1/1 -> Sum4/1
  Fcn/1 -> Product1/1
  Sum4/1 -> Switch3/1
  Fcn3/1 -> roughness correction1/1
  Mach/1 -> roughness correction/2, Fcn4/1, roughness correction1/2, Fcn3/1, Fcn/1, Fcn2/1, c21/1, c2/2, Switch3/2, Switch1/2, c1/2, Fcn1/1
  Fcn4/1 -> roughness correction1/3
  roughness correction1/1 -> roughness correction/1
  roughness correction/1 -> Gain1/1
  Sum3/1 -> Divide/2, Sum1/1, Reynolds/2

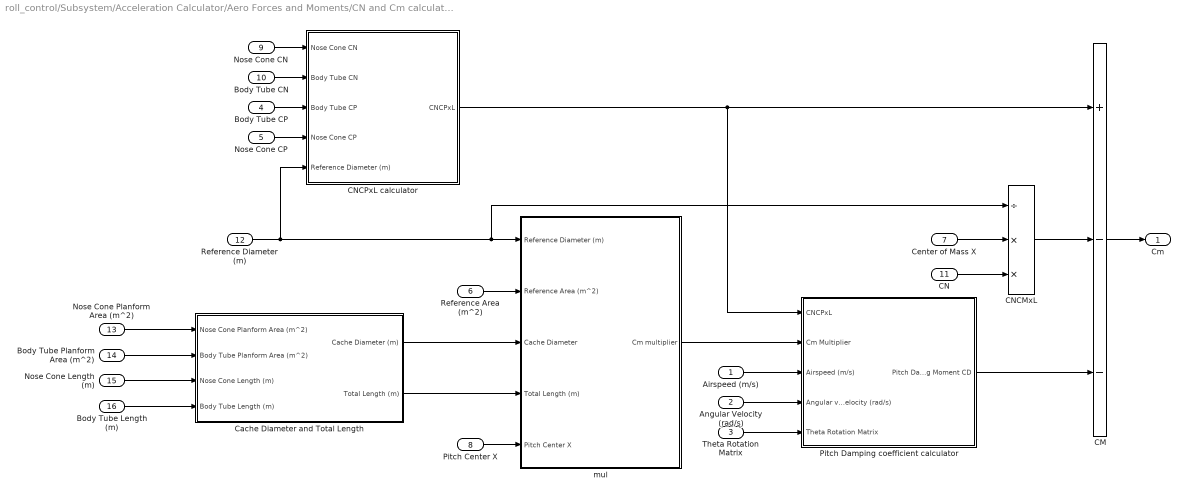
== system roll_control/Subsystem/Acceleration Calculator/Aero Forces and Moments/CN and Cm calculator/CM calculator ==
  Airspeed (m/s) : Inport
  Angular Velocity (rad/s) : Inport  Port=2
  Theta Rotation Matrix : Inport  Port=3
  Body Tube CP : Inport  Port=4
  Nose Cone CP : Inport  Port=5
  Reference Area (m^2) : Inport  Port=6
  Center of Mass X : Inport  Port=7
  Pitch Center X : Inport  Port=8
  Nose Cone CN : Inport  Port=9
  Body Tube CN : Inport  Port=10
  CN : Inport  Port=11
  Reference Diameter (m) : Inport  Port=12
  Nose Cone Planform Area (m^2) : Inport  Port=13
  Body Tube Planform Area (m^2) : Inport  Port=14
  Nose Cone Length (m) : Inport  Port=15
  Body Tube Length (m) : Inport  Port=16
  CM : Sum  Inputs=+--
  CNCMxL : Product  Inputs=/**
  CNCPxL calculator : Subsystem
  Cache Diameter and Total Length : Subsystem
  Pitch Damping coefficient calculator : Subsystem
  mul : Subsystem
  Cm : Outport  VectorParamsAs1DForOutWhenUnconnected=off
  wires:
  CNCPxL calculator/1("CNCPxL ") -> Pitch Damping coefficient calculator/1(CNCPxL), CM/1
  Pitch Center X/1 -> mul/5(Pitch Center X)
  Cache Diameter and Total Length/2(Total Length (m)) -> mul/4(Total Length (m))
  Reference Diameter (m)/1 -> CNCMxL/1, mul/1(Reference Diameter (m)), CNCPxL calculator/5(Reference Diameter (m))
  Nose Cone CP/1 -> CNCPxL calculator/4(Nose Cone CP)
  CM/1 -> Cm/1
  Body Tube CP/1 -> CNCPxL calculator/3(Body Tube CP)
  Cache Diameter and Total Length/1(Cache Diameter (m)) -> mul/3(Cache Diameter)
  mul/1(Cm multiplier) -> Pitch Damping coefficient calculator/2(Cm Multiplier)
  Angular Velocity (rad/s)/1 -> Pitch Damping coefficient calculator/4(Angular velocity (rad/s))
  Airspeed (m/s)/1 -> Pitch Damping coefficient calculator/3(Airspeed (m/s))
  Reference Area (m^2)/1 -> mul/2(Reference Area (m^2))
  Theta Rotation Matrix/1 -> Pitch Damping coefficient calculator/5(Theta Rotation Matrix)
  Body Tube CN/1 -> CNCPxL calculator/2(Body Tube CN)
  Nose Cone CN/1 -> CNCPxL calculator/1(Nose Cone CN)
  Nose Cone Planform Area (m^2)/1 -> Cache Diameter and Total Length/1(Nose Cone Planform Area (m^2))
  Body Tube Planform Area (m^2)/1 -> Cache Diameter and Total Length/2(Body Tube Planform Area (m^2))
  Nose Cone Length (m)/1 -> Cache Diameter and Total Length/3(Nose Cone Length (m))
  Body Tube Length (m)/1 -> Cache Diameter and Total Length/4(Body Tube Length (m))
  Center of Mass X/1 -> CNCMxL/2
  CN/1 -> CNCMxL/3
  Pitch Damping coefficient calculator/1(Pitch Damping Moment CD) -> CM/3
  CNCMxL/1 -> CM/2

== system roll_control/Subsystem/Acceleration Calculator/Aero Forces and Moments/CN and Cm calculator/CN calculator ==
  Reference Area (m^2) : Inport
  AoA (rads) : Inport  Port=2
  Mach : Inport  Port=3
  Nose Cone Planform Area (m^2) : Inport  Port=4
  Body Tube Planform Area (m^2) : Inport  Port=5
  CN multiplier : Subsystem
  Component CN : Subsystem
  Normal Force CD : Sum
  Nose Cone CN : Outport  VectorParamsAs1DForOutWhenUnconnected=off
  Body Tube CN : Outport  Port=2  VectorParamsAs1DForOutWhenUnconnected=off
  CN : Outport  Port=3  VectorParamsAs1DForOutWhenUnconnected=off
  wires:
  Mach/1 -> CN multiplier/2(Mach)
  CN multiplier/1(CN multiplier) -> Component CN/2(CN multiplier)
  Component CN/1(Nose Cone CN) -> Normal Force CD/1, Nose Cone CN/1
  AoA (rads)/1 -> CN multiplier/1(AoA (rads)), Component CN/1(AoA (rads))
  Nose Cone Planform Area (m^2)/1 -> Component CN/4(Nose Cone Planform Area)
  Component CN/2(Body Tube CN) -> Normal Force CD/2, Body Tube CN/1
  Body Tube Planform Area (m^2)/1 -> Component CN/5(Body Tube Planform Area)
  Reference Area (m^2)/1 -> Component CN/3(Reference Area)
  Normal Force CD/1 -> CN/1

== system roll_control/Subsystem/Acceleration Calculator/Aero Forces and Moments/CN and Cm calculator/CM calculator/CNCPxL calculator ==
  Nose Cone CN : Inport
  Body Tube CN : Inport  Port=2
  Body Tube CP : Inport  Port=3
  Nose Cone CP : Inport  Port=4
  Reference Diameter (m) : Inport  Port=5
  Add1 : Sum
  CNCPxL : Product  Inputs=*/
  CNCPxL1 : Product  Inputs=*/
  CNCPxL2 : Product  Inputs=*/
  Product1 : Product
  Product3 : Product
  "CNCPxL " : Outport  VectorParamsAs1DForOutWhenUnconnected=off
  wires:
  Product1/1 -> Add1/1, CNCPxL2/1
  CNCPxL/1 -> "CNCPxL "/1
  Nose Cone CN/1 -> Product1/1
  Reference Diameter (m)/1 -> CNCPxL2/2, CNCPxL1/2, CNCPxL/2
  Body Tube CN/1 -> Product3/1
  Add1/1 -> CNCPxL/1
  Body Tube CP/1 -> Product3/2
  Product3/1 -> CNCPxL1/1, Add1/2
  Nose Cone CP/1 -> Product1/2

== system roll_control/Subsystem/Acceleration Calculator/Aero Forces and Moments/CN and Cm calculator/CM calculator/Cache Diameter and Total Length ==
  Nose Cone Planform Area (m^2) : Inport
  Body Tube Planform Area (m^2) : Inport  Port=2
  Nose Cone Length (m) : Inport  Port=3
  Body Tube Length (m) : Inport  Port=4
  Cache Diameter : Product  Inputs=*/
  Total Length : Sum
  Total Planform Area : Sum
  Cache Diameter (m) : Outport  VectorParamsAs1DForOutWhenUnconnected=off
  Total Length (m) : Outport  Port=2  VectorParamsAs1DForOutWhenUnconnected=off
  wires:
  Total Planform Area/1 -> Cache Diameter/1
  Nose Cone Planform Area (m^2)/1 -> Total Planform Area/1
  Body Tube Length (m)/1 -> Total Length/2
  Nose Cone Length (m)/1 -> Total Length/1
  Body Tube Planform Area (m^2)/1 -> Total Planform Area/2
  Total Length/1 -> Total Length (m)/1, Cache Diameter/2
  Cache Diameter/1 -> Cache Diameter (m)/1

== system roll_control/Subsystem/Acceleration Calculator/Aero Forces and Moments/CN and Cm calculator/CM calculator/Pitch Damping coefficient calculator ==
  CNCPxL : Inport
  Cm Multiplier : Inport  Port=2
  Airspeed (m/s) : Inport  Port=3
  Angular velocity (rad/s) : Inport  Port=4
  Theta Rotation Matrix : Inport  Port=5
  Dot Product3 : DotProduct  SaturateOnIntegerOverflow=on  OutDataTypeStr=Inherit: Inherit via internal rule
  Math Function6 : Math  Operator=square  SignedPower=on  SaturateOnIntegerOverflow=on
  MinMax : MinMax  Inputs=2
  Multiply : Product  Inputs=**/
  Pitch DampingMoment CD : Product
  Pitch Rate : Product  Inputs=*/  Multiplication=Matrix(*)
  Sel6 : Selector  InputPortWidth=3  IndexOptions=Index vector (dialog)  Indices=2  OutputSizes=1
  Sign : Signum
  Pitch Damping Moment CD : Outport  VectorParamsAs1DForOutWhenUnconnected=off
  wires:
  Dot Product3/1 -> Multiply/3
  Airspeed (m/s)/1 -> Dot Product3/2, Dot Product3/1
  Sign/1 -> Pitch DampingMoment CD/1
  CNCPxL/1 -> MinMax/1
  Math Function6/1 -> Multiply/2
  Multiply/1 -> MinMax/2
  Pitch DampingMoment CD/1 -> Pitch Damping Moment CD/1
  Sel6/1 -> Sign/1, Math Function6/1
  MinMax/1 -> Pitch DampingMoment CD/2
  Theta Rotation Matrix/1 -> Pitch Rate/2
  Cm Multiplier/1 -> Multiply/1
  Pitch Rate/1 -> Sel6/1
  Angular velocity (rad/s)/1 -> Pitch Rate/1

== system roll_control/Subsystem/Acceleration Calculator/Aero Forces and Moments/CN and Cm calculator/CM calculator/mul ==
  Reference Diameter (m) : Inport
  Reference Area (m^2) : Inport  Port=2
  Cache Diameter : Inport  Port=3
  Total Length (m) : Inport  Port=4
  Pitch Center X : Inport  Port=5
  Add : Sum
  Add2 : Sum  Inputs=+-
  Constant2 : Constant  Value=4
  Gain2 : Gain  Gain=3 * 0.275
  Math Function : Math  Operator=pow  SignedPower=on  SaturateOnIntegerOverflow=on
  Math Function1 : Math  Operator=pow  SignedPower=on  SaturateOnIntegerOverflow=on
  Multiply : Product  Inputs=**//
  Cm multiplier : Outport  VectorParamsAs1DForOutWhenUnconnected=off
  wires:
  Math Function1/1 -> Add/2
  Pitch Center X/1 -> Add2/2, Math Function1/1
  Constant2/1 -> Math Function/2, Math Function1/2
  Add/1 -> Multiply/1
  Math Function/1 -> Add/1
  Reference Area (m^2)/1 -> Multiply/4
  Multiply/1 -> Gain2/1
  Add2/1 -> Math Function/1
  Reference Diameter (m)/1 -> Multiply/3
  Gain2/1 -> Cm multiplier/1
  Total Length (m)/1 -> Add2/1
  Cache Diameter/1 -> Multiply/2

== system roll_control/Subsystem/Acceleration Calculator/Aero Forces and Moments/CN and Cm calculator/CN calculator/CN multiplier ==
  AoA (rads) : Inport
  Mach : Inport  Port=2
  1 : Constant
  Compare To Constant : simulink/Logic and Bit Operations/Compare To Constant  relop=<  const=.05  OutDataTypeStr=boolean
  Compare To Constant1 : simulink/Logic and Bit Operations/Compare To Constant  relop=>  const=pi/4  OutDataTypeStr=boolean
  Gain : Gain  Gain=1/0.05
  Logical Operator : Logic  AllPortsSameDT=off  OutDataTypeStr=boolean
  Square : Math  Operator=square  SignedPower=on  SaturateOnIntegerOverflow=on
  cnmul : Switch  Criteria=u2 > Threshold
  CN multiplier : Outport  VectorParamsAs1DForOutWhenUnconnected=off
  wires:
  AoA (rads)/1 -> Compare To Constant1/1
  Logical Operator/1 -> cnmul/2
  Compare To Constant/1 -> Logical Operator/2
  Mach/1 -> Compare To Constant/1, Gain/1
  Compare To Constant1/1 -> Logical Operator/1
  Square/1 -> cnmul/1
  1/1 -> cnmul/3
  Gain/1 -> Square/1
  cnmul/1 -> CN multiplier/1

== system roll_control/Subsystem/Acceleration Calculator/Aero Forces and Moments/CN and Cm calculator/CN calculator/Component CN ==
  AoA (rads) : Inport
  CN multiplier : Inport  Port=2
  Reference Area : Inport  Port=3
  Nose Cone Planform Area : Inport  Port=4
  Body Tube Planform Area : Inport  Port=5
  Add : Sum
  BodyTube CN : Product
  Constant : Constant  Value=2
  Divide2 : Product  Inputs=**/
  Gain1 : Gain  Gain=1.1
  NoseCone CN : Product
  Product1 : Product
  Product2 : Product
  Trigonometric Function : Trigonometry
  Nose Cone CN : Outport  VectorParamsAs1DForOutWhenUnconnected=off
  Body Tube CN : Outport  Port=2  VectorParamsAs1DForOutWhenUnconnected=off
  wires:
  Body Tube Planform Area/1 -> Product1/2
  NoseCone CN/1 -> Nose Cone CN/1
  Constant/1 -> Add/1
  Nose Cone Planform Area/1 -> Product2/1
  Add/1 -> NoseCone CN/2
  BodyTube CN/1 -> Body Tube CN/1
  CN multiplier/1 -> Divide2/2
  AoA (rads)/1 -> Trigonometric Function/1
  Divide2/1 -> Gain1/1
  Reference Area/1 -> Divide2/3
  Gain1/1 -> Product2/2, Product1/1
  Product2/1 -> Add/2
  Trigonometric Function/1 -> Divide2/1, BodyTube CN/2, NoseCone CN/1
  Product1/1 -> BodyTube CN/1

== matlab function roll_control/Affine LQR (New LQR at every x seconds) Position/MATLAB Function1 ==
  settings: updateMethod=DISCRETE
  data: state input; u input; K_x_out output; time input; k_0_out output; Thrust_magnitude input
function [K_x_out, k_0_out] = fcn(state, u, time, Thrust_magnitude)
  coder.extrinsic('affine_controller_position'); 
  persistent last_time K_x k_0

  if Thrust_magnitude < 0.1
    Thrust = 0.1;
  else
    Thrust = Thrust_magnitude;
  end
  
  if isempty(last_time)
    last_time = 0;
    K_x = zeros(3, 10);
    k_0 = zeros(3, 1);
    [K_x, k_0, ~] = affine_controller_position(state, u, inf, Thrust);
  end
  
  if time - last_time > 0.1
    [K_x, k_0, ~] = affine_controller_position(state, u, inf, Thrust);
  end
  
  K_x_out = K_x;
  k_0_out = k_0;
  
  last_time = time;
end

== matlab function roll_control/Tracker/MATLAB Function1 ==
  settings: updateMethod=DISCRETE
  data: state input; u input; K_x_out output; time input; k_0_out output; Thrust_magnitude input; x_d input; u_d input
function [K_x_out, k_0_out] = fcn(state, u, time, Thrust_magnitude, x_d, u_d)
  coder.extrinsic('affine_controller_position'); 
  persistent last_time K_x k_0
  
  if isempty(last_time)
    last_time = 0;
    K_x = zeros(3, 10);
    k_0 = zeros(3, 1);
    [K_x, k_0, ~] = Tracker(state, u, 3.45, Thrust_magnitude, x_d, u_d);
  end
  
  if time >= 3.45
    return
  end
  
  if time - last_time > 0.1
    [K_x, k_0, ~] = Tracker(state, u, 3.45 - time, Thrust_magnitude, x_d, u_d);
  end
  
  K_x_out = K_x;
  k_0_out = k_0;
  
  last_time = time;
end

== matlab function roll_control/Subsystem4/Desired Quaternion ==
  settings: updateMethod=DISCRETE
  data: current_direction input; Desired_Direction input; Error_Quaternion output size=[1 4]
function Error_Quaternion  = func(current_direction, Desired_Direction)
    w = cross(current_direction, Desired_Direction);
    q = [dot(current_direction, Desired_Direction),w]; 
    Error_Quaternion = normalize([q(1) + norm(q), q(2:4)]);

== matlab function roll_control/Subsystem4/Desired Quaternion1 ==
  settings: updateMethod=DISCRETE
  data: Desired_Direction input; a output size=[1 4]
function a  = func(Desired_Direction)
    m = sqrt(2 + 2 * Desired_Direction(3));
    w = (1 / m) * [-Desired_Direction(2) Desired_Direction(1) 0];
    a =  [0.5 * m, w];

== matlab function roll_control/Affine LQR (New LQR at every x seconds)/MATLAB Function1 ==
  settings: updateMethod=DISCRETE
  data: state input; u input; K_x_out output; time input; k_0_out output
function [K_x_out, k_0_out] = fcn(state, u, time)
  coder.extrinsic('affine_controller'); 
  persistent last_time K_x k_0

  if isempty(last_time)
    last_time = 0;
    K_x = zeros(3, 9);
    k_0 = zeros(3, 1);
%     [K_x, k_0, t, ~] = affine_controller(state, u, 3.45 - time);
    [K_x, k_0, ~] = affine_controller(state, u, inf);
  end
  
  if time - last_time > 10
%     [K_x, k_0, t, ~] = affine_controller(state, u, 3.45 - time);
    [K_x, k_0, ~] = affine_controller(state, u, inf);
  end
  
%   [ ~, ix ] = min( abs( t - (time - last_time) ) );
%   
%   K_x_out = K_x(:, :, ix);
%   k_0_out = k_0(:, :, ix);
  K_x_out = K_x;
  k_0_out = k_0;
  
  last_time = time;
end

== matlab function roll_control/MATLAB Function2 ==
  data: Inertia input; state input; u input; estimated_state output; ThrustTable input; time input; masscgI input
function estimated_state = fcn(Inertia, state, u, ThrustTable, time, masscgI)
  coder.extrinsic('NonlinearStateEstimationForActuatorDelay'); 
  estimated_state = zeros(15, 1);
  estimated_state = NonlinearStateEstimationForActuatorDelay(Inertia, state, u, ThrustTable, time, 0, masscgI);
end

== matlab function roll_control/MATLAB Function3 ==
  data: time input; final_state output; state input
function final_state = fcn(time, state)
  coder.extrinsic('RunNonlinearStateEstimationForActuatorDelay')
  final_state = zeros(16, 1);
  Moments_t = [0 3.45]';
  Moments_data = [0 0 0; 0 0 0];
  Moments = [Moments_t Moments_data];
  final_state = RunNonlinearStateEstimationForActuatorDelay(time, state, Moments);
end
